simulink model "rad2radpi"  (Simulink 5.0)
settings: Solver=ode45  StartTime=0.0  StopTime=100.0  RelTol=1e-3
libraries: simulink x2
settings Model: LastModifiedBy=Roger  OutputOption=SpecifiedOutputTimes  OutputTimes=[0:.01:100]

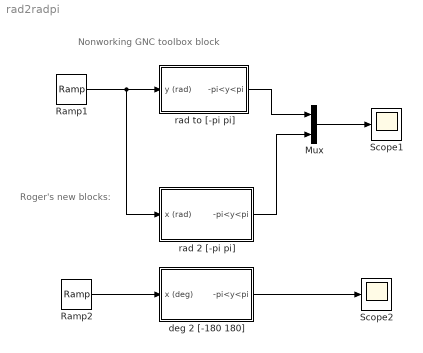
== system rad2radpi ==
  note: Nonworking
      | GNC toolbox block
  note: Roger's new blocks:
  Mux : Mux  Inputs=2
  Ramp1 : simulink/Sources/Ramp  slope=20*pi/180  start=0  X0=-4*pi
  Ramp2 : simulink/Sources/Ramp  slope=20  start=0  X0=-4*180
  Scope1 : Scope
      settings: TimeRange=100  YMin=-10  YMax=20
  Scope2 : Scope
      settings: TimeRange=100  YMin=-200  YMax=200
  deg 2 [-180 180] : Subsystem  Description=|
      | % Routine that maps an angle in degrees into [-180, 180).
      | % Roger Skjetne - 05.09.2003
      mask Description:
      | % Routine that maps an angle in degrees into [-180, 180).
      | % Roger Skjetne - 05.09.2003
  rad 2 [-pi pi] : Subsystem  Description=|
      | % Routine that maps an angle in radians into [-pi, pi).
      | % Roger Skjetne - 05.09.2003
      mask Description:
      | % Program that maps an angle in radians into [-pi, pi).
      | % Roger Skjetne - 05.09.2003
  rad to [-pi pi] : Subsystem  AncestorBlock=MarineGNC/Library blocks/Angle conversion/rad to [-pi pi]
  wires:
  Ramp1/1 -> rad to [-pi pi]/1(y (rad)), rad 2 [-pi pi]/1(x (rad))
  rad to [-pi pi]/1(-pi<y<pi) -> Mux/1
  rad 2 [-pi pi]/1(-pi<y<pi) -> Mux/2
  Mux/1 -> Scope1/1
  Ramp2/1 -> deg 2 [-180 180]/1(x (deg))
  deg 2 [-180 180]/1(-pi<y<pi) -> Scope2/1

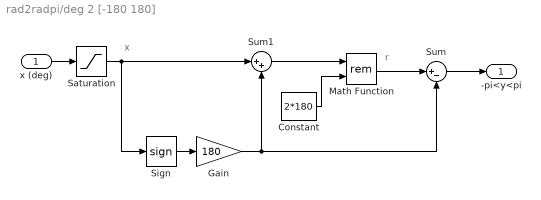
== system rad2radpi/deg 2 [-180 180] ==
  note: r
  note: x
  x (deg) : Inport
  Constant : Constant  Value=2*180
  Gain : Gain  Gain=180  SaturateOnIntegerOverflow=on
  Math Function : Math  Operator=rem
  Saturation : Saturate  UpperLimit=1e10  LowerLimit=-1e10
  Sign : Signum
  Sum : Sum  Inputs=|+-  SaturateOnIntegerOverflow=on
  Sum1 : Sum  Inputs=|++  SaturateOnIntegerOverflow=on
  -pi<y<pi : Outport
  wires:
  Sum/1 -> -pi<y<pi/1
  Math Function/1 -> Sum/1
  Constant/1 -> Math Function/2
  Sum1/1 -> Math Function/1
  Gain/1 -> Sum1/2, Sum/2
  Sign/1 -> Gain/1
  x (deg)/1 -> Saturation/1
  Saturation/1 -> Sign/1, Sum1/1

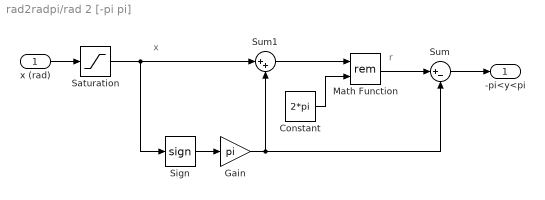
== system rad2radpi/rad 2 [-pi pi] ==
  note: x
  note: r
  x (rad) : Inport
  Constant : Constant  Value=2*pi
  Gain : Gain  Gain=pi  SaturateOnIntegerOverflow=on
  Math Function : Math  Operator=rem
  Saturation : Saturate  UpperLimit=1e10  LowerLimit=-1e10
  Sign : Signum
  Sum : Sum  Inputs=|+-  SaturateOnIntegerOverflow=on
  Sum1 : Sum  Inputs=|++  SaturateOnIntegerOverflow=on
  -pi<y<pi : Outport
  wires:
  x (rad)/1 -> Saturation/1
  Sign/1 -> Gain/1
  Gain/1 -> Sum/2, Sum1/2
  Sum1/1 -> Math Function/1
  Constant/1 -> Math Function/2
  Math Function/1 -> Sum/1
  Sum/1 -> -pi<y<pi/1
  Saturation/1 -> Sum1/1, Sign/1

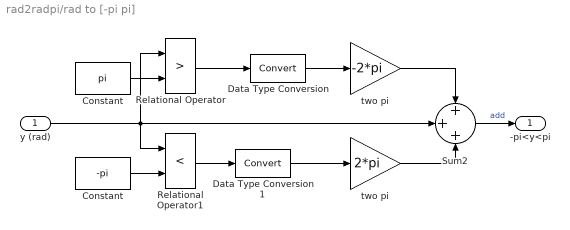
== system rad2radpi/rad to [-pi pi] ==
  y (rad) : Inport
  Constant : Constant  Value=pi
  "Constant " : Constant  Value=-pi
  Data Type Conversion : DataTypeConversion  DataType=double  SaturateOnIntegerOverflow=on
  Data Type Conversion1 : DataTypeConversion  DataType=double  SaturateOnIntegerOverflow=on
  Relational Operator : RelationalOperator  Operator=>  InputSameDT=on
  Relational Operator1 : RelationalOperator  Operator=<  InputSameDT=on
  Sum2 : Sum  Inputs=+++  SaturateOnIntegerOverflow=on  InputSameDT=on
  two pi : Gain  Gain=-2*pi  SaturateOnIntegerOverflow=on
  "two pi  " : Gain  Gain=2*pi  SaturateOnIntegerOverflow=on
  -pi<y<pi : Outport  InitialOutput=0
  wires:
  Data Type Conversion1/1 -> "two pi  "/1
  Data Type Conversion/1 -> two pi/1
  y (rad)/1 -> Relational Operator/1, Relational Operator1/1, Sum2/2
  Sum2/1 -> -pi<y<pi/1  "add"
  "two pi  "/1 -> Sum2/3
  two pi/1 -> Sum2/1
  Relational Operator1/1 -> Data Type Conversion1/1
  "Constant "/1 -> Relational Operator1/2
  Relational Operator/1 -> Data Type Conversion/1
  Constant/1 -> Relational Operator/2
